simulink model "smart_parking_v1"  (R2019a)
settings: Solver=FixedStepAuto  StartTime=0.0  StopTime=inf  RelTol=1e-3  EnableMultiTasking=on
libraries: arduinolib x5, LCDlib x1
settings Model: SimulationMode=external  ExtModeTrigDuration=2  Creator=User  LastModifiedBy=Shyam lal
settings OptimizationCC: EnhancedBackFolding=on  PassReuseOutputArgsAs=Individual arguments  MaxStackSize=64  OptimizeBlockOrder=speed  DifferentSizesBufferReuse=on  OptimizationCustomize=off
settings DebuggingCC: ParameterTunabilityLossMsg=error  ArithmeticOperatorsInVariantConditions=warning
settings HardwareCC: ProdBitPerInt=16  ProdBitPerPointer=16  ProdBitPerSizeT=16  ProdBitPerPtrDiffT=16  ProdLargestAtomicFloat=None  ProdWordSize=8  ProdHWDeviceType=Atmel->AVR
settings SFSimCC: MATLABDynamicMemAlloc=off
settings RTWCC: SystemTargetFile=ert.tlc  HardwareBoard=Arduino Uno  TLCOptions=-aInlineSetEventsForThisBaseRateFcn=TLC_FALSE -aSuppressMultiTaskScheduler=TLC_FALSE -aRateBasedStepFcn=1  TemplateMakefile=ert_default_tmf  GenerateReport=on  Toolchain=Arduino AVR  BuildConfiguration=Faster Runs  IncludeHyperlinkInReport=on  LaunchReport=on  GenerateTraceInfo=on  GenerateTraceReport=on  GenerateTraceReportSl=on  GenerateTraceReportSf=on  GenerateTraceReportEml=on
settings CodeAppCC: ForceParamTrailComments=on  IgnoreCustomStorageClasses=off  OperatorAnnotations=on  SimulinkDataObjDesc=on  SFDataObjDesc=on  InsertBlockDesc=on
settings ERTTargetCC: SupportContinuousTime=on  SupportVariableSizeSignals=on  ExtModeStaticAllocSize=250

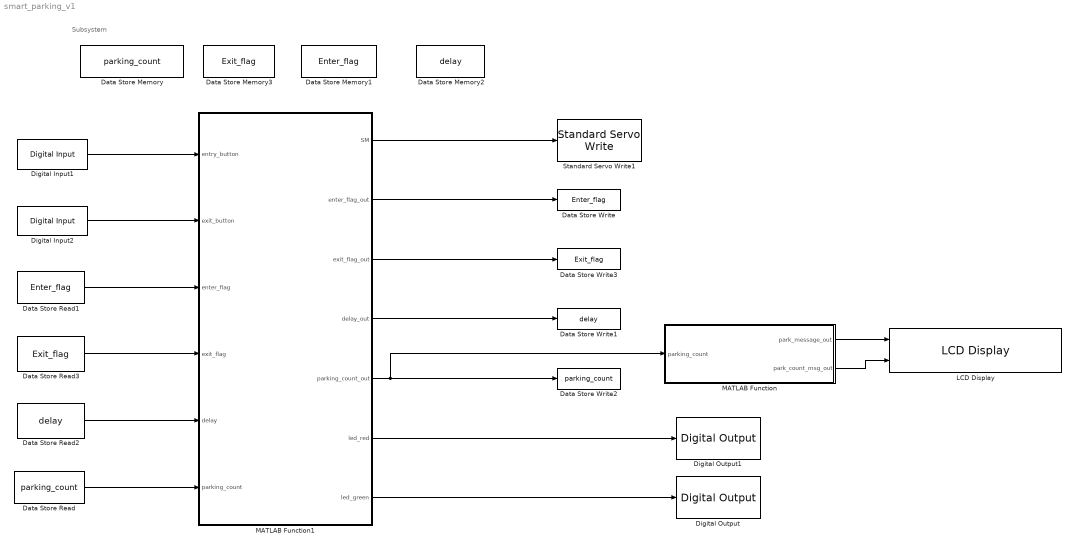
== system smart_parking_v1 ==
  note: Subsystem
  Data Store Memory : DataStoreMemory  DataStoreName=parking_count  ReadBeforeWriteMsg=warning  WriteAfterWriteMsg=warning  WriteAfterReadMsg=warning  InitialValue=3  ShowAdditionalParam=off
  Data Store Memory1 : DataStoreMemory  DataStoreName=Enter_flag  ReadBeforeWriteMsg=warning  WriteAfterWriteMsg=warning  WriteAfterReadMsg=warning  ShowAdditionalParam=off
  Data Store Memory2 : DataStoreMemory  DataStoreName=delay  ReadBeforeWriteMsg=warning  WriteAfterWriteMsg=warning  WriteAfterReadMsg=warning  InitialValue=2  ShowAdditionalParam=off
  Data Store Memory3 : DataStoreMemory  DataStoreName=Exit_flag  ReadBeforeWriteMsg=warning  WriteAfterWriteMsg=warning  WriteAfterReadMsg=warning  ShowAdditionalParam=off
  Data Store Read : DataStoreRead  DataStoreName=parking_count
  Data Store Read1 : DataStoreRead  DataStoreName=Enter_flag
  Data Store Read2 : DataStoreRead  DataStoreName=delay
  Data Store Read3 : DataStoreRead  DataStoreName=Exit_flag
  Data Store Write : DataStoreWrite  DataStoreName=Enter_flag
  Data Store Write1 : DataStoreWrite  DataStoreName=delay
  Data Store Write2 : DataStoreWrite  DataStoreName=parking_count
  Data Store Write3 : DataStoreWrite  DataStoreName=Exit_flag
  Digital Input1 : arduinolib/Digital Input  pinNumber=13  sampleTime=1  blockPlatform=arduino
      settings: SourceProductName=Simulink Support Package for Arduino Hardware
  Digital Input2 : arduinolib/Digital Input  pinNumber=10  sampleTime=1  blockPlatform=arduino
      settings: SourceProductName=Simulink Support Package for Arduino Hardware
  Digital Output : arduinolib/Digital Output  pinNumber=8  blockPlatform=arduino
  Digital Output1 : arduinolib/Digital Output  pinNumber=9  blockPlatform=arduino
  LCD Display : LCDlib/LCD Display  pins=[12, 11, 5, 4, 3, 2]
      settings: SourceProductName=LCD Library
  MATLAB Function : MATLAB Function  TreatAsAtomicUnit=on
  MATLAB Function1 : MATLAB Function  TreatAsAtomicUnit=on
  Standard Servo Write1 : arduinolib/Standard Servo Write  pinNumber=6  ServoIndex=0  blockPlatform=arduino
      settings: SourceProductName=Simulink Support Package for Arduino Hardware
  wires:
  MATLAB Function1/1(SM) -> Standard Servo Write1/1
  MATLAB Function1/2(enter_flag_out) -> Data Store Write/1
  Data Store Read1/1 -> MATLAB Function1/3(enter_flag)
  Data Store Read2/1 -> MATLAB Function1/5(delay)
  MATLAB Function1/4(delay_out) -> Data Store Write1/1
  Data Store Read/1 -> MATLAB Function1/6(parking_count)
  MATLAB Function1/5(parking_count_out) -> MATLAB Function/1(parking_count), Data Store Write2/1
  MATLAB Function/2(park_count_msg_out) -> LCD Display/2
  MATLAB Function/1(park_message_out) -> LCD Display/1
  Digital Input1/1 -> MATLAB Function1/1(entry_button)
  Digital Input2/1 -> MATLAB Function1/2(exit_button)
  Data Store Read3/1 -> MATLAB Function1/4(exit_flag)
  MATLAB Function1/3(exit_flag_out) -> Data Store Write3/1
  MATLAB Function1/7(led_green) -> Digital Output/1
  MATLAB Function1/6(led_red) -> Digital Output1/1

== matlab function smart_parking_v1/MATLAB Function1 ==
  data: SM output; entry_button input; exit_button input; enter_flag input; exit_flag input; enter_flag_out output; exit_flag_out output; delay input; delay_out output; parking_count input; parking_count_out output; led_red output; led_green output
function [SM,enter_flag_out,exit_flag_out,delay_out,parking_count_out,led_red,led_green] = fcn(entry_button,exit_button,enter_flag,exit_flag,delay, parking_count)
if entry_button 
    enter_flag_out=1;
    exit_flag_out=0;
elseif exit_button
    exit_flag_out=1;
    enter_flag_out=0;
else
    enter_flag_out=enter_flag;
    exit_flag_out=exit_flag;
end
if enter_flag || enter_flag_out
    if delay>0
        if parking_count > 0
            delay_out=delay-1;
            parking_count_out= parking_count;
            led_green=1;
            led_red=0;
            SM=[90];
        else
            delay_out=delay;
            parking_count_out= parking_count;
            led_green=0;
            led_red=1;
            SM=[0];
        end
    else
        if parking_count > 0
            parking_count_out = parking_count - 1;
            SM=[0];
        else
            parking_count_out = parking_count;
            SM=[0];
        end
        enter_flag_out=0;
        delay_out=2;
        led_red=1;
        led_green=0;
    end
elseif exit_flag || exit_flag_out
    if delay>0
        if parking_count < 3
            delay_out=delay-1;
            parking_count_out= parking_count;
            led_green=1;
            led_red=0;
            SM=[90];
        else
            delay_out=delay;
            parking_count_out= parking_count;
            led_green=0;
            led_red=1;
            SM=[0];
        end
    else
        if parking_count < 3
            parking_count_out = parking_count +1;
            SM=[0];
        else
            parking_count_out = parking_count;
            SM=[0];
        end
        exit_flag_out=0;
        delay_out=2;
        led_red=1;
        led_green=0;
    end  
else
    SM=[0];
    delay_out=delay;
    enter_flag_out=enter_flag;
    exit_flag_out=exit_flag;
    parking_count_out= parking_count;
    led_red=1;
    led_green=0;
end
end

== matlab function smart_parking_v1/MATLAB Function ==
  data: park_message_out output; parking_count input; park_count_msg_out output
function [park_message_out,park_count_msg_out] = fcn(parking_count)
if parking_count > 0
    park_message_out = [[87],[69],[76],[67],[79],[77],[69],[33],[33],[33],[32],[32],[32],[32]];  
 else
    park_message_out  = [[80],[76],[90],[32],[67],[79],[77],[69],[32],[76],[65],[84],[69],[82]];
 end
switch parking_count
        case 0
            park_count_msg_out=[[78],[111],[32],[111],[102],[32],[83],[108],[111],[116],[115],[58],[48],[48]];
        case 1
            park_count_msg_out=[[78],[111],[32],[111],[102],[32],[83],[108],[111],[116],[115],[58],[48],[49]];
        case 2
            park_count_msg_out=[[78],[111],[32],[111],[102],[32],[83],[108],[111],[116],[115],[58],[48],[50]];
        case 3
            park_count_msg_out=[[78],[111],[32],[111],[102],[32],[83],[108],[111],[116],[115],[58],[48],[51]];
        case 4
            park_count_msg_out=[[78],[111],[32],[111],[102],[32],[83],[108],[111],[116],[115],[58],[48],[52]];
        case 5
            park_count_msg_out=[[78],[111],[32],[111],[102],[32],[83],[108],[111],[116],[115],[58],[48],[53]];
        case 6
            park_count_msg_out=[[78],[111],[32],[111],[102],[32],[83],[108],[111],[116],[115],[58],[48],[54]];
        case 7
            park_count_msg_out=[[78],[111],[32],[111],[102],[32],[83],[108],[111],[116],[115],[58],[48],[55]];
        case 8
            park_count_msg_out=[[78],[111],[32],[111],[102],[32],[83],[108],[111],[116],[115],[58],[48],[56]];
        case 9
            park_count_msg_out=[[78],[111],[32],[111],[102],[32],[83],[108],[111],[116],[115],[58],[48],[57]];
        case 10
            park_count_msg_out=[[78],[111],[32],[111],[102],[32],[83],[108],[111],[116],[115],[58],[49],[48]];
        case 11
            park_count_msg_out=[[78],[111],[32],[111],[102],[32],[83],[108],[111],[116],[115],[58],[49],[49]];
        case 12
            park_count_msg_out=[[78],[111],[32],[111],[102],[32],[83],[108],[111],[116],[115],[58],[49],[50]];
        case 13
            park_count_msg_out=[[78],[111],[32],[111],[102],[32],[83],[108],[111],[116],[115],[58],[49],[51]];  
        otherwise
            park_count_msg_out=[[78],[111],[32],[111],[102],[32],[83],[108],[111],[116],[115],[58],[69],[82]];
 end
end
